simulink model "Data_driven_MPC_ScheduledData"  (R2020b)
settings: Solver=FixedStepAuto  StartTime=0.0  StopTime=T_sim  FixedStep=dt  RelTol=1e-3
values from neighbouring files (symbols this model uses):
  A_alpha1 = [ones(1,N-L+1) zeros(1,(m+p)*L+m+p+p*L+1)]    [Init_FixedData.m]    (also in Init_ScheduledData.m; Init_UpdatedData.m)
  A_init = [zeros(nu*m,N-L+1) eye(nu*m) zeros(nu*m,m*(L-nu)+p*L+m+p+p*L+1) ... (first row only)    [Init_FixedData.m]    (also in Init_ScheduledData.m; Init_UpdatedData.m)
  A_TEC = [zeros((nu+1)*m,N-L+1) zeros((nu+1)*m,m*(L-nu-1)) eye((nu+1)*m) zeros((nu+1)*m,p*L) -repmat(eye(m),nu+1,1) zeros(m*(nu+1),p+p*L+1) ... (first row only)    [Init_FixedData.m]    (also in Init_ScheduledData.m; Init_UpdatedData.m)
  Adyn_e = A_dyn    [Init_ScheduledData.m]
  Adyn_t = A_dyn    [Init_ScheduledData.m]
  b_alpha1 = 1    [Init_FixedData.m]    (also in Init_ScheduledData.m; Init_UpdatedData.m)
  b_dyn = zeros((m+p)*L,1)    [Init_FixedData.m]    (also in Init_ScheduledData.m; Init_UpdatedData.m)
  b_TEC = zeros((m+p)*(nu+1),1)    [Init_FixedData.m]    (also in Init_ScheduledData.m; Init_UpdatedData.m)
  dt = 0.1    [Init_FixedData.m]    (also in Init_ScheduledData.m; Init_UpdatedData.m)
  H_e = H    [Init_ScheduledData.m]
  H_t = H    [Init_ScheduledData.m]
  L = L_true + nu    (= 56)    [Init_FixedData.m]    (also in Init_ScheduledData.m; Init_UpdatedData.m)
  lambda_beta = 0    [Init_FixedData.m]    (also in Init_ScheduledData.m; Init_UpdatedData.m)
  lb = [-inf*ones(N-L+1,1); repmat(u_min,L,1); repmat(y_min,L,1); us_min; y_min; -inf*ones(p*L,1); -inf]    [Init_FixedData.m]    (also in Init_ScheduledData.m = [-inf*ones(N-L+1,1); repmat(u_min,L,1); repmat(y_min,L,1); u; Init_UpdatedData.m)
  m = 2    [DataGen.m]    (also in Init_FixedData.m; Init_ScheduledData.m; Init_UpdatedData.m)
  N = size(ud,2)    [Init_FixedData.m]    (also in Init_ScheduledData.m = 311; Init_UpdatedData.m)
  NOISE = false    [Init_FixedData.m]    (also in Init_ScheduledData.m = 0; Init_UpdatedData.m = 0)
  noise_bound_cl = 1*pi/180    (= 0.0174532925199)    [Init_FixedData.m]    (also in Init_ScheduledData.m; Init_UpdatedData.m)
  nu = 6    [Init_FixedData.m]    (also in Init_ScheduledData.m; Init_UpdatedData.m)
  p = 3    [DataGen.m]    (also in Init_FixedData.m; Init_ScheduledData.m; Init_UpdatedData.m)
  Sy_e = S_y    [Init_ScheduledData.m]
  Sy_t = S_y    [Init_ScheduledData.m]
  T_Track = 5    [Init_FixedData.m]    (also in Init_ScheduledData.m; Init_UpdatedData.m)
  T_Track2 = 20    [Init_FixedData.m]    (also in Init_ScheduledData.m; Init_UpdatedData.m)
  T_Track3 = 30    [Init_FixedData.m]    (also in Init_ScheduledData.m; Init_UpdatedData.m)
  ub = [inf*ones(N-L+1,1) ; repmat(u_max,L,1); repmat(y_max,L,1); us_max; y_max;  inf*ones(p*L,1);  inf]    [Init_FixedData.m]    (also in Init_ScheduledData.m = [inf*ones(N-L+1,1) ; repmat(u_max,L,1); repmat(y_max,L,1); u; Init_UpdatedData.m)
  x0 = [0/180*pi; 0; 0/180*pi; 0; 0; 0]    [DataGen.m]    (also in Init_FixedData.m = [0*pi/180; 0; -30*pi/180; 0; 0; 0;]; Init_ScheduledData.m = [0*pi/180; 0; -30*pi/180; 0; 0; 0;]; Init_UpdatedData.m = [0*pi/180; 0; -30*pi/180; 0; 0; 0;])
  y_T1 = [0*pi/180; 0*pi/180; 0]    [Init_FixedData.m]    (also in Init_ScheduledData.m; Init_UpdatedData.m)
  y_T2 = [90*pi/180; 0*pi/180; 0]    [Init_FixedData.m]    (also in Init_ScheduledData.m; Init_UpdatedData.m)
  y_T3 = [0*pi/180; 0*pi/180; 0]    [Init_FixedData.m]    (also in Init_ScheduledData.m; Init_UpdatedData.m)
  y_T4 = [0*pi/180; -30*pi/180; 0]    [Init_FixedData.m]    (also in Init_ScheduledData.m; Init_UpdatedData.m)
libraries: simulink x5
settings Model: Creator=Fabian  LastModifiedBy=Fabian

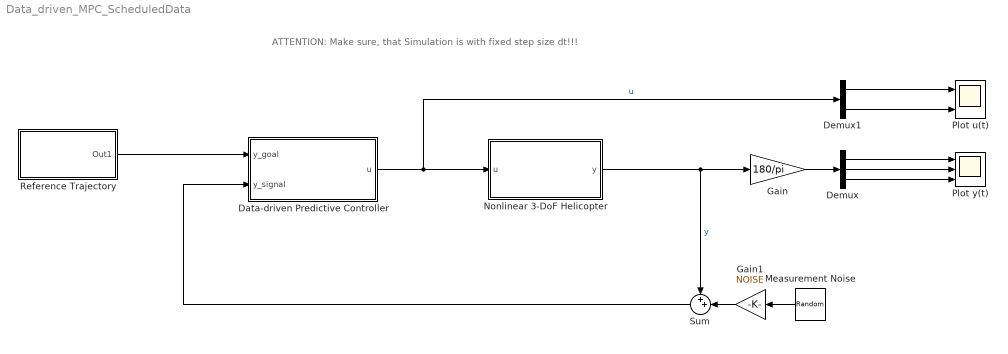
== system Data_driven_MPC_ScheduledData ==
  note: ATTENTION: Make sure, that Simulation is with fixed step size dt!!!
  Data-driven Predictive Controller : Subsystem
  Demux : Demux  Outputs=3
  Demux1 : Demux  Outputs=2
  Gain : Gain  Gain=180/pi
  Gain1 : Gain  Gain=NOISE
  Measurement Noise : UniformRandomNumber  Minimum=-noise_bound_cl  Maximum=noise_bound_cl  Seed=[3;4;5]  SampleTime=dt
  Nonlinear 3-DoF Helicopter : Subsystem
  Plot u(t) : Scope  NumInputPorts=2
  Plot y(t) : Scope  NumInputPorts=3
  Reference Trajectory : Subsystem
  Sum : Sum  Inputs=++|
  wires:
  Reference Trajectory/1(Out1) -> Data-driven Predictive Controller/1(y_goal)
  Demux1/2 -> Plot u(t)/2
  Demux/1 -> Plot y(t)/1
  Demux/2 -> Plot y(t)/2
  Nonlinear 3-DoF Helicopter/1(y) -> Gain/1, Sum/1  "y"
  Gain/1 -> Demux/1
  Demux/3 -> Plot y(t)/3
  Data-driven Predictive Controller/1(u) -> Demux1/1, Nonlinear 3-DoF Helicopter/1(u)  "u"
  Gain1/1 -> Sum/2
  Sum/1 -> Data-driven Predictive Controller/2(y_signal)
  Measurement Noise/1 -> Gain1/1
  Demux1/1 -> Plot u(t)/1

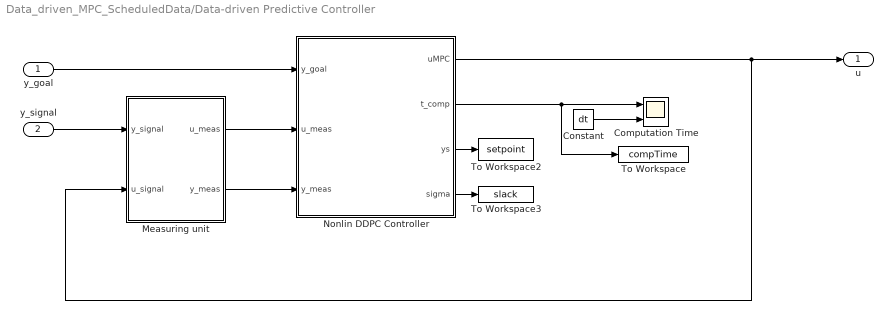
== system Data_driven_MPC_ScheduledData/Data-driven Predictive Controller ==
  y_goal : Inport
  y_signal : Inport  Port=2
  Computation Time : Scope  NumInputPorts=2
  Constant : Constant  Value=dt
  Measuring unit : Subsystem
  Nonlin DDPC Controller : MATLAB Function  TreatAsAtomicUnit=on
  To Workspace : ToWorkspace  VariableName=compTime  SaveFormat=Timeseries  SampleTime=-1
  To Workspace2 : ToWorkspace  VariableName=setpoint  SaveFormat=Timeseries  SampleTime=-1
  To Workspace3 : ToWorkspace  VariableName=slack  SaveFormat=Timeseries  SampleTime=-1
  u : Outport
  wires:
  y_signal/1 -> Measuring unit/1(y_signal)
  Measuring unit/1(u_meas) -> Nonlin DDPC Controller/2(u_meas)
  Measuring unit/2(y_meas) -> Nonlin DDPC Controller/3(y_meas)
  Nonlin DDPC Controller/1(uMPC) -> Measuring unit/2(u_signal), u/1
  Nonlin DDPC Controller/2(t_comp) -> Computation Time/1, To Workspace/1
  Constant/1 -> Computation Time/2
  y_goal/1 -> Nonlin DDPC Controller/1(y_goal)
  Nonlin DDPC Controller/3(ys) -> To Workspace2/1
  Nonlin DDPC Controller/4(sigma) -> To Workspace3/1

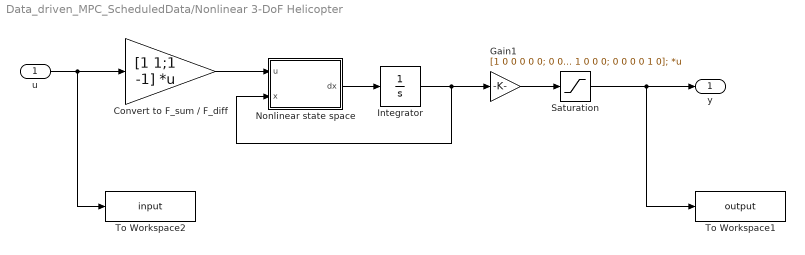
== system Data_driven_MPC_ScheduledData/Nonlinear 3-DoF Helicopter ==
  u : Inport
  Convert to F_sum / F_diff : Gain  Gain=[1 1;1 -1]  Multiplication=Matrix(K*u)
  Gain1 : Gain  Gain=[1 0 0 0 0 0; 0 0 1 0 0 0; 0 0 0 0 1 0];  Multiplication=Matrix(K*u)
  Integrator : Integrator  InitialCondition=x0
  Nonlinear state space : MATLAB Function  TreatAsAtomicUnit=on
  Saturation : Saturate  UpperLimit=[inf; 33*pi/180; 90*pi/180]  LowerLimit=[-inf; -33*pi/180; -90*pi/180]
  To Workspace1 : ToWorkspace  VariableName=output  SaveFormat=Timeseries  SampleTime=-1
  To Workspace2 : ToWorkspace  VariableName=input  SaveFormat=Timeseries  SampleTime=-1
  y : Outport
  wires:
  Nonlinear state space/1(dx) -> Integrator/1
  Integrator/1 -> Gain1/1, Nonlinear state space/2(x)
  u/1 -> To Workspace2/1, Convert to F_sum / F_diff/1
  Convert to F_sum / F_diff/1 -> Nonlinear state space/1(u)
  Gain1/1 -> Saturation/1
  Saturation/1 -> To Workspace1/1, y/1

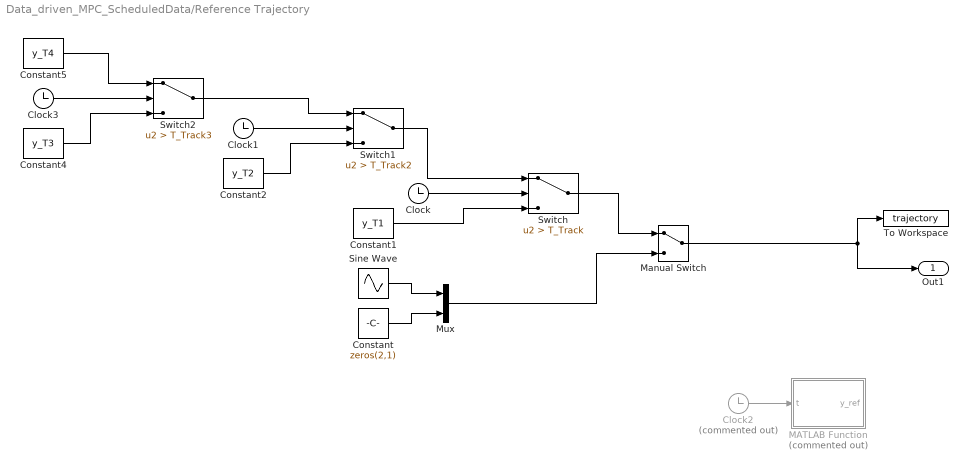
== system Data_driven_MPC_ScheduledData/Reference Trajectory ==
  Clock : Clock
  Clock1 : Clock
  Clock2 : Clock  Commented=on
  Clock3 : Clock
  Constant : Constant  Value=zeros(2,1)
  Constant1 : Constant  Value=y_T1
  Constant2 : Constant  Value=y_T2
  Constant4 : Constant  Value=y_T3
  Constant5 : Constant  Value=y_T4
  MATLAB Function : MATLAB Function  Commented=on  TreatAsAtomicUnit=on
  Manual Switch : ManualSwitch
  Mux : Mux  Inputs=2
  Sine Wave : Sin  Amplitude=45*pi/180  Frequency=2*pi*1/25  Phase=-5*2*pi*1/25  SampleTime=0
  Switch : Switch  Criteria=u2 > Threshold  Threshold=T_Track
  Switch1 : Switch  Criteria=u2 > Threshold  Threshold=T_Track2
  Switch2 : Switch  Criteria=u2 > Threshold  Threshold=T_Track3
  To Workspace : ToWorkspace  VariableName=trajectory  SaveFormat=Timeseries  SampleTime=-1
  Out1 : Outport
  wires:
  Manual Switch/1 -> Out1/1, To Workspace/1
  Switch2/1 -> Switch1/1
  Mux/1 -> Manual Switch/2
  Constant2/1 -> Switch1/3
  Clock1/1 -> Switch1/2
  Clock/1 -> Switch/2
  Sine Wave/1 -> Mux/1
  Constant/1 -> Mux/2
  Switch/1 -> Manual Switch/1
  Switch1/1 -> Switch/1
  Constant1/1 -> Switch/3
  Clock2/1 -> MATLAB Function/1(t)
  Clock3/1 -> Switch2/2
  Constant5/1 -> Switch2/1
  Constant4/1 -> Switch2/3

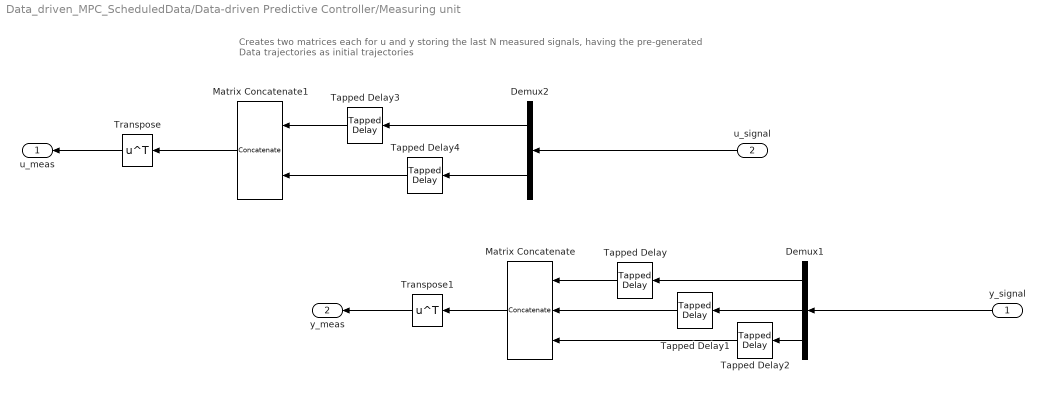
== system Data_driven_MPC_ScheduledData/Data-driven Predictive Controller/Measuring unit ==
  note: Creates two matrices each for u and y storing the last N measured signals,
      | having the pre-generated Data trajectories as initial trajectories
  y_signal : Inport
  u_signal : Inport  Port=2
  Demux1 : Demux  Outputs=3
  Demux2 : Demux  Outputs=2
  Matrix Concatenate : Concatenate  NumInputs=3  Mode=Multidimensional array  ConcatenateDimension=2
  Matrix Concatenate1 : Concatenate  Mode=Multidimensional array  ConcatenateDimension=2
  Tapped Delay : simulink/Discrete/Tapped Delay  vinit=x0(1)*ones(nu,1)  samptime=-1  NumDelays=nu  DelayOrder=Oldest  includeCurrent=off
  Tapped Delay1 : simulink/Discrete/Tapped Delay  vinit=x0(3)*ones(nu,1)  samptime=-1  NumDelays=nu  DelayOrder=Oldest  includeCurrent=off
  Tapped Delay2 : simulink/Discrete/Tapped Delay  vinit=x0(5)*ones(nu,1)  samptime=-1  NumDelays=nu  DelayOrder=Oldest  includeCurrent=off
  Tapped Delay3 : simulink/Discrete/Tapped Delay  vinit=0  samptime=-1  NumDelays=nu  DelayOrder=Oldest  includeCurrent=off
  Tapped Delay4 : simulink/Discrete/Tapped Delay  vinit=0  samptime=-1  NumDelays=nu  DelayOrder=Oldest  includeCurrent=off
  Transpose : Math  Operator=transpose  SaturateOnIntegerOverflow=on
  Transpose1 : Math  Operator=transpose  SaturateOnIntegerOverflow=on
  u_meas : Outport
  y_meas : Outport  Port=2
  wires:
  Demux2/2 -> Tapped Delay4/1
  Demux2/1 -> Tapped Delay3/1
  Tapped Delay3/1 -> Matrix Concatenate1/1
  Demux1/1 -> Tapped Delay/1
  Demux1/2 -> Tapped Delay1/1
  Tapped Delay4/1 -> Matrix Concatenate1/2
  Demux1/3 -> Tapped Delay2/1
  Tapped Delay1/1 -> Matrix Concatenate/2
  Tapped Delay/1 -> Matrix Concatenate/1
  Tapped Delay2/1 -> Matrix Concatenate/3
  u_signal/1 -> Demux2/1
  y_signal/1 -> Demux1/1
  Matrix Concatenate1/1 -> Transpose/1
  Transpose/1 -> u_meas/1
  Matrix Concatenate/1 -> Transpose1/1
  Transpose1/1 -> y_meas/1

== matlab function Data_driven_MPC_ScheduledData/Reference Trajectory/MATLAB Function ==
  data: t input; y_ref output
function y_ref = fcn(t)
       

    y_home_v = [0*pi/180; 0*pi/180; 0];  
    y_cargo_v = [90*pi/180; 0*pi/180; 0]; 
    y_cargo = [90*pi/180; -22*pi/180; 0];
    y_drop_v = [450*pi/180; 0*pi/180; 0];
    y_drop = [450*pi/180; -22*pi/180; 0];
    y_home = [0*pi/180; -27*pi/180; 0];

    if (0 <= t) && t < 5
        y_ref = y_home_v;
    elseif (5 <= t) && t < 17
        y_ref = y_cargo_v;
    elseif (17 <= t) && t < 30
        y_ref = y_cargo;
    elseif (30 <= t) && t < 35
        y_ref = y_cargo_v;
    elseif (35 <= t) && t < 50
        y_ref = y_drop_v;
    elseif (50 <= t) && t < 65
        y_ref = y_drop;
    elseif (65 <= t) && t < 70
        y_ref = y_drop_v;
    elseif (70 <= t) && t < 90
        y_ref = y_home_v;
    elseif t > 90
        y_ref = y_home;
    else
        y_ref = y_home;
    end

end

== matlab function Data_driven_MPC_ScheduledData/Nonlinear 3-DoF Helicopter/Nonlinear state space ==
  data: u input; x input; dx output
function dx = fcn(u,x)

%%%%%%%%%%%%%%%%%%%%%%%%%%%%%%%%%%%%%%%%%%%%%%%%%%%%%%%%%%%%%%%%%%%%%%%%
%%%%%%%%%%%%%%%%%%%%% ATTENTION %%%%%%%%%%%%%%%%%%%%%%%%%%%%%%%%%%%%%%%%
%%%% Input is F_sum and F_diff, not F_front and F_back !! %%%%%%%%%%%%%%
%%%%%%%%%%%%%%%%%%%%%%%%%%%%%%%%%%%%%%%%%%%%%%%%%%%%%%%%%%%%%%%%%%%%%%%%

    m_H = 1.322;
    m_A = 2.638;

    Jxx = 1.1455;
    Jyy = 1.1184;
    Jzz = 0.032;

    r = 0.1775;

    rHx = -0.089;
    rHz = 0.655;
    rAHx = -0.034;
    rAHz = 0.0193;

    g = 9.81;
    
    dalph = x(2);
    bet = x(3);
    dbet = x(4);
    gam = x(5);
    dgam = x(6);
    
    Fsum = u(1);
    Fdiff = u(2);
    
    dx = [dalph;...
     1/Jxx * Fsum*sin(gam) * (rHx*sin(bet) - rHz*cos(bet));...
     dbet;...
     1/Jyy * (-(m_A+m_H)*g *(rAHz*cos(bet) - rAHx*sin(bet)) + Fsum * rHz*cos(gam));...
     dgam;...
     -1/Jzz * r * Fdiff];

end

== matlab function Data_driven_MPC_ScheduledData/Data-driven Predictive Controller/Nonlin DDPC Controller ==
  data: y_goal input; u_meas input; uMPC output; y_meas input; t_comp output; lb parameter; ub parameter; b_dyn parameter; A_init parameter; b_TEC parameter; b_alpha1 parameter; A_TEC parameter; A_alpha1 parameter; m parameter; p parameter; N parameter; L parameter; nu parameter; lambda_beta parameter; ys output; sigma output; H_t parameter; H_e parameter; Adyn_t parameter; Adyn_e parameter; Sy_t parameter; Sy_e parameter
function [uMPC, t_comp, ys, sigma] = fcn(y_goal, u_meas, y_meas, lb, ub, b_dyn, A_init, b_TEC, b_alpha1, A_TEC, A_alpha1, m, p, N, L, nu, lambda_beta, H_t, H_e, Adyn_t, Adyn_e, Sy_t, Sy_e)

    % Data-driven Model Predictive Control using Nonlinear Data with
    % scheduled data update during the control process
    
    % ATTENTION: Simulation Step Size must be dt (fixed)!!!
    
    t_begin = tic; %Track computation time
    
    %% Setup Quadprog
    
    %Quadprog setup
    %(Simulink coder only allows for 'Active-set' algorithm)
    coder.extrinsic('quadprog');
    options = optimoptions('quadprog','Algorithm','active-set','Display','Off');
    
    %% Update Init Data
    
    % Take past nu measurements for init
    u_init = u_meas(:);
    y_init = y_meas(:);
        
    b_init = [u_init(:); y_init(:)];
    
    %% Schedule data
    
    travel = 1;
    if y_goal(2) < 0
        travel = 0;
    end
    
    %% Set up and solve Main Quadratic Program 
    
    uMPC = zeros(2,1); 
    sol_0 = zeros(N-L+1+(m+p)*L+m+p+p*L+1,1);
    
    if travel
        % Travel taks, use respective data and parameters
        
        % Include tracking point y_goal
        f = [zeros(N-L+1,1);zeros((m+p)*L+m,1);-2*Sy_t*y_goal;zeros(p*L,1);-lambda_beta];
        
        A_eq = [Adyn_t; A_init; A_TEC; A_alpha1];
        b_eq = [b_dyn ; b_init; b_TEC; b_alpha1];

        A_ineq = [];
        b_ineq = [];

        %Solving QP
        [sol,~,~,~,~] = quadprog(H_t,f,A_ineq,b_ineq,A_eq,b_eq,lb,ub,sol_0,options);
    else
        % Elevation taks, use respective data and parameters
        
        % Include tracking point y_goal
        f = [zeros(N-L+1,1);zeros((m+p)*L+m,1);-2*Sy_e*y_goal;zeros(p*L,1);-lambda_beta];
        
        A_eq = [Adyn_e; A_init; A_TEC; A_alpha1];
        b_eq = [b_dyn ; b_init; b_TEC; b_alpha1];

        A_ineq = [];
        b_ineq = [];

        %Solving QP
        [sol,~,~,~,~] = quadprog(H_e,f,A_ineq,b_ineq,A_eq,b_eq,lb,ub,sol_0,options);
    end
    
    %Extract solution
    u_sol = sol(N-L+1+1:N-L+1+m*L);
    uMPC = u_sol(nu*m+1:nu*m+m);
    
    %%%%%%%% ATTENTION: uMPC is Front and Backmotor Force %%%%%%%%%%%%%%%%%
    
    %% Yield numeric measures
    
    t_comp = toc(t_begin);
    
    %% Yield artificial setpoint
    
    ys = zeros(3,1);
    ys = sol((N-L+1)+(m+p)*L+m+1 : (N-L+1)+(m+p)*L+m+p);
    
    %% Yield slack
    
    sig_size = p*L;
    sigma_vec = zeros(sig_size,1);
    sigma_vec = sol(N-L+1+(m+p)*L+m+p+1:N-L+1+(m+p)*L+m+p+p*L);
    sigma = norm(sigma_vec);
   
end
